simulink model "sfunction"  (R2022b)
settings: Solver=VariableStepAuto  StartTime=0.0  StopTime=2  RelTol=1e-3
libraries: slpidlib x1
settings Model: Creator=ericliu  LastModifiedBy=Lenovo
settings OptimizationCC: ReuseModelBlockBuffer=on
settings RTWCC: GPUComputeCapability=5.0

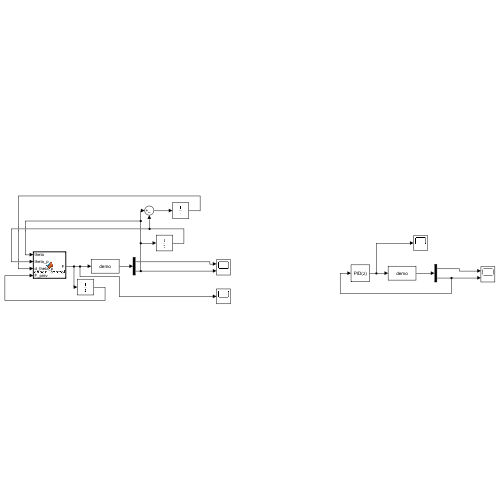
[thumbnail: Simulink's stored preview of the top-level diagram]
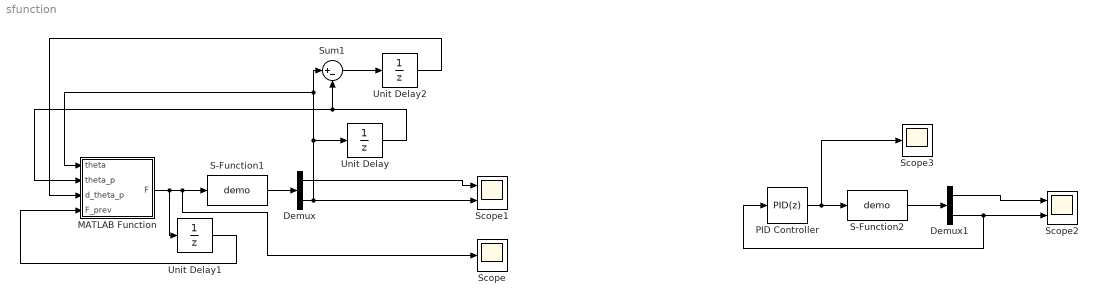
== system sfunction ==
  Demux : Demux  Outputs=2
  Demux1 : Demux  Outputs=2
  MATLAB Function : MATLAB Function  TreatAsAtomicUnit=on
  PID Controller : slpidlib/PID Controller  Controller=PID  Form=Parallel  TimeDomain=Discrete-time  UseExternalTs=off  SampleTime=0.0001  IntegratorMethod=Forward Euler  FilterMethod=Forward Euler  ControllerParametersSource=internal  P=200  I=0.001  UseKiTs=off  D=10  N=100  UseFilter=on  TunerSelectOption=Transfer Function Based (PID Tuner App)  InitialConditionSource=internal  InitialConditionForIntegrator=0  InitialConditionForFilter=0  DifferentiatorICPrevScaledInput=0  ExternalReset=none  TrackingMode=off  Kt=1  LimitOutput=off  SatLimitsSource=internal  UpperSaturationLimit=inf  LowerSaturationLimit=-inf  LinearizeAsGain=on  AntiWindupMode=none  Kb=1  LimitIntegrator=off  UpperIntegratorSaturationLimit=inf  LowerIntegratorSaturationLimit=-inf  POutMin=[]  POutMax=[]  IOutMin=[]  IOutMax=[]  DOutMin=[]  DOutMax=[]  NOutMin=[]  NOutMax=[]  SumOutMin=[]  SumOutMax=[]  SaturationOutMin=[]  SaturationOutMax=[]  PParamMin=[]  PParamMax=[]  IParamMin=[]  IParamMax=[]  DParamMin=[]  DParamMax=[]  NParamMin=[]  NParamMax=[]  KbParamMin=[]  KbParamMax=[]  KtParamMin=[]  KtParamMax=[]  KbOutMin=[]  KbOutMax=[]  KtOutMin=[]  KtOutMax=[]  IntegratorOutMin=[]  IntegratorOutMax=[]  FilterOutMin=[]  FilterOutMax=[]  SumI1OutMin=[]  SumI1OutMax=[]  SumI2OutMin=[]  SumI2OutMax=[]  SumI3OutMin=[]  SumI3OutMax=[]  SumI4OutMin=[]  SumI4OutMax=[]  SumDOutMin=[]  SumDOutMax=[]  DifferentiatorOutMin=[]  DifferentiatorOutMax=[]  FilterDiffOutCoefMin=[]  FilterDiffOutCoefMax=[]  ReciprocalOutMin=[]  ReciprocalOutMax=[]  SumDenOutMin=[]  SumDenOutMax=[]  SumNumOutMin=[]  SumNumOutMax=[]  DivideOutMin=[]  DivideOutMax=[]  UdiffTsProdOutMin=[]  UdiffTsProdOutMax=[]  NTsProdOutMin=[]  NTsProdOutMax=[]  UintegralTsProdOutMin=[]  UintegralTsProdOutMax=[]  UngainTsProdOutMin=[]  UngainTsProdOutMax=[]  ClampingZeroOutDataTypeStr=Inherit: Inherit via back propagation  ClampingZeroOutMin=[]  ClampingZeroOutMax=[]  FilterDenConstantOutDataTypeStr=Inherit: Inherit via back propagation  FilterDenConstantOutMin=[]  FilterDenConstantOutMax=[]  PCopyOutDataTypeStr=Inherit: Inherit via back propagation  PCopyOutMin=[]  PCopyOutMax=[]  NCopyOutDataTypeStr=Inherit: Inherit via back propagation  NCopyOutMin=[]  NCopyOutMax=[]  IntegratorContinuousStateAttributes=''  IntegratorStateMustResolveToSignalObject=off  IntegratorRTWStateStorageClass=Auto  FilterContinuousStateAttributes=''  FilterStateMustResolveToSignalObject=off  FilterRTWStateStorageClass=Auto  ParallelPVariant=InternalParameters  IdealPVariant=Disabled  IVariant=InternalParameters  DVariant=InternalParameters  IntegratorVariant=Discrete  SatVariant=Disabled  AWVariant=Passthrough  PCopyVariant=Disabled  TRVariant=Disabled  FdbkBlocksVariant=Forward  IdealPFdbkVariant=Disabled  SatFdbkVariant=Disabled  DerivativeFilterVariant=ForwardEulerFilter  NVariant=InternalParameters  NCopyVariant=Disabled  FilterICVariant=InternalICsFilter  IntegratorICVariant=InternalICs  ExternalResetVariant=Disabled  TRSumVariant=Passthrough  SumFdbkVariant=Disabled  SumVariant=Sum_PID  TsampFilterVariant=InternalTs  TsampNgainVariant=Passthrough  TsampIntegralVariant=Passthrough  ExternalSaturationOutDataTypeStr=Inherit: Same as second input
  S-Function1 : S-Function  FunctionName=demo  SFunctionDeploymentMode=off  EnableBusSupport=off
  S-Function2 : S-Function  FunctionName=demo  SFunctionDeploymentMode=off  EnableBusSupport=off
  Scope : Scope
  Scope1 : Scope  NumInputPorts=2
  Scope2 : Scope  NumInputPorts=2
  Scope3 : Scope
  Sum1 : Sum  Inputs=|+-
  Unit Delay : UnitDelay  SampleTime=0.0001  HasFrameUpgradeWarning=on
  Unit Delay1 : UnitDelay  SampleTime=0.0001  HasFrameUpgradeWarning=on
  Unit Delay2 : UnitDelay  SampleTime=0.0001  HasFrameUpgradeWarning=on
  wires:
  MATLAB Function/1(F) -> Unit Delay1/1, Scope/1, S-Function1/1
  Demux/1 -> Scope1/1
  Unit Delay/1 -> MATLAB Function/2(theta_p), Sum1/2
  Unit Delay1/1 -> MATLAB Function/4(F_prev)
  S-Function1/1 -> Demux/1
  Demux/2 -> Unit Delay/1, Sum1/1, MATLAB Function/1(theta), Scope1/2
  Sum1/1 -> Unit Delay2/1
  Unit Delay2/1 -> MATLAB Function/3(d_theta_p)
  S-Function2/1 -> Demux1/1
  Demux1/2 -> PID Controller/1, Scope2/2
  Demux1/1 -> Scope2/1
  PID Controller/1 -> Scope3/1, S-Function2/1

== matlab function sfunction/MATLAB Function ==
  data: theta input; theta_p input; d_theta_p input; F output; F_prev input
function F = expert_control(theta, theta_p, d_theta_p, F_prev)
    % 专家控制函数，计算当前的控制力 F
    % 输入参数：
    %   theta: 当前角度（当前时刻的角度）
    %   theta_p: 上一时刻的角度
    %   d_theta_p: 上一时刻的角速度（角度变化率）
    %   F_prev: 上一时刻的控制力

    % 定义常数（增益和阈值）
    Kp = 200;   % 比例增益
    Ti = 0.001; % 积分时间常数
    Td = 10;    % 微分时间常数
    T = 0.0001; % 采样时间

  % 原始参数
  theta1 = 0.1; % 阈值 θ1
  theta2 = 0.3; % 阈值 θ2
  thetam = 0.5; % 阈值 θm

%     % 角度阈值（用于判断不同的控制策略）
%     theta1 = 0.1; % 阈值 θ1，表示小角度区间
%     theta2 = 0.6; % 阈值 θ2，表示中等角度区间
%     thetam = 0.8; % 阈值 θm，表示大角度区间

    % 稳定角度设定
    theta_d = 0; % 稳定角度，期望角度通常设为0

  Ks = 1;    % 专家控制增益 Ks
  Kb = 1.3;  % 专家控制增益 Kb
  Fm = 25;   % 最大控制力 Fm

%     % 专家控制增益和最大控制力
%     Ks = 1.5;    % 专家控制增益 Ks（当在小角度区域时使用）
%     Kb = 1.8;    % 专家控制增益 Kb（当在大角度区域时使用）
%     Fm = 200;    % 最大控制力 Fm（当角度足够大时使用最大控制力）

    % 初始化增益 K
    K = 0;
    
    % 计算当前角度增量
    delta_theta = theta - theta_p;  % 当前角度与上时刻角度的差
    abs_theta = abs(theta);         % 当前角度的绝对值，用于判断在哪个区间

    % 根据不同角度区间选择控制策略
    if abs_theta >= thetam
        % 规则 1：|θ(k)| ≥ θm（大角度情况）
        % 当角度大于阈值 θm 时，直接输出最大控制力，且方向与角度方向相同
        F = sign(theta) * Fm;  % 根据角度的符号输出最大控制力
        return;  % 直接返回，不再继续计算

    elseif abs_theta >= theta2 && abs_theta < thetam
        % 规则 2：θ2 ≤ |θ(k)| < θm（中等角度情况）
        % 当角度在 θ2 和 θm 之间时，使用不同的增益 K 来调整控制力
        if theta * delta_theta > 0
            K = Kb;  % 规则 2-1：角度与增量同方向时，使用较大增益 Kb
        elseif theta * delta_theta < 0
            if delta_theta * d_theta_p > 0
                K = 1;  % 规则 2-2a：角度与增量反向，且增量加速时使用较小增益 1
            elseif delta_theta * d_theta_p < 0
                K = Kb; % 规则 2-2b：角度与增量反向，且增量减速时使用较大增益 Kb
            end
        end

    elseif abs_theta >= theta1 && abs_theta < theta2
        % 规则 3：θ1 ≤ |θ(k)| < θ2（小角度到中等角度情况）
        % 当角度在 θ1 和 θ2 之间时，使用不同的增益 K 来调整控制力
        if theta * delta_theta > 0
            K = 1;  % 规则 3-1：角度与增量同方向时，使用增益 1
        elseif theta * delta_theta < 0
            if delta_theta * d_theta_p > 0
                K = Ks; % 规则 3-2a：角度与增量反向，且增量加速时使用较小增益 Ks
            elseif delta_theta * d_theta_p < 0
                K = 1;  % 规则 3-2b：角度与增量反向，且增量减速时使用增益 1
            end
        end

    elseif abs_theta < theta1
        % 规则 4：|θ(k)| < θ1（非常小的角度）
        % 当角度非常小，使用增益K来保持控制平稳
        K = 1;
    end

    % 使用增量型离散 PID 控制计算当前的控制力
    % 当前控制力由上一个时刻的控制力 F_prev 和增量型 PID 控制公式计算得出
    F = F_prev + K * (Kp * delta_theta + T / Ti * (theta - theta_d) + Td / T * (delta_theta - d_theta_p) );
end
